simulink model "laser"  (R2017b)
settings: Solver=VariableStepAuto  StartTime=0.0  StopTime=10.0  RelTol=1e-3
values from neighbouring files (symbols this model uses):
  Amp0d = [1]    [System.m]    (also in System_submitted.m = [Amp0d1 Amp0d0])
  Amp0n = [1]    [System.m]    (also in System_submitted.m = Amp0n0)
  Amp1d = Amp0d    [System.m]    (also in SystemHeadless.m; System_submitted.m)
  Amp1n = Amp0n    [System.m]    (also in SystemHeadless.m; System_submitted.m)
  AmpSat0 = MotorParam(NomV)    [System.m]    (also in SystemHeadless.m = q0(NomV); System_submitted.m = q0(NomV))
  AmpSat1 = Big    [System.m]    (also in SystemHeadless.m = AmpSat0; System_submitted.m = AmpSat0)
  BackEMF0 = 1/K_B    [System.m]    (also in SystemHeadless.m = 1 / q0(SpdK); System_submitted.m = 1 / q0(SpdK))
  BackEMF1 = 1/K_B1    [System.m]    (also in SystemHeadless.m = 1 / q1(SpdK); System_submitted.m = 1 / q1(SpdK))
  Distance = 1    [CONSTANTS.m]
  Elec0d = [L_a R_a]    [System.m]    (also in SystemHeadless.m = [Elec0d1, Elec0d0]; System_submitted.m = [Elec0d1, Elec0d0])
  Elec0n = [1]    [System.m]    (also in SystemHeadless.m = 1; System_submitted.m = 1)
  Elec1d = [L_a R_a]    [System.m]    (also in SystemHeadless.m = [Elec1d1, Elec1d0]; System_submitted.m = [Elec1d1, Elec1d0])
  Elec1n = [1]    [System.m]    (also in SystemHeadless.m = 1; System_submitted.m = 1)
  JntSat1 = JntLim * RadPerDeg    [System.m]    (also in SystemHeadless.m = joint_limit; System_submitted.m = joint_limit)
  Mech0d = [J_system F_kf 0]    [System.m]    (also in SystemHeadless.m = [J_0, B_0, K_0]; System_submitted.m = [J_0, B_0, K_0])
  Mech0n = [1 0]    [System.m]    (also in SystemHeadless.m = [1, 0]; System_submitted.m = [1, 0])
  Mech1d = [J_rotor F_kf 0]    [System.m]    (also in SystemHeadless.m = [J_1, B_1, K_1]; System_submitted.m = [J_1, B_1, K_1])
  Mech1n = [1 0]    [System.m]    (also in SystemHeadless.m = [1, 0]; System_submitted.m = [1, 0])
  NomI0 = MotorParam(NomCurr)    [System.m]    (also in System_submitted.m = q0(NomCurr))
  NomI1 = MotorParam(NomCurr)    [System.m]    (also in System_submitted.m = q1(NomCurr))
  Sens0 = SensV / (SensAng * RadPerDeg)    [System.m]    (also in SystemHeadless.m; System_submitted.m)
  Sens1 = SensV / (SensAng * RadPerDeg)    [System.m]    (also in SystemHeadless.m; System_submitted.m)
  StallI0 = MotorParam(StallCurr)    [System.m]    (also in System_submitted.m = q0(StallCurr))
  StallI1 = MotorParam(StallCurr)    [System.m]    (also in System_submitted.m = q1(StallCurr))
  StFric0 = F_sf    [System.m]    (also in SystemHeadless.m = mu_SF * inner_fg; System_submitted.m = mu_SF * inner_fg)
  TConst0 = K_T    [System.m]    (also in SystemHeadless.m = q0(TorqueK); System_submitted.m = q0(TorqueK))
  TConst1 = K_T1    [System.m]    (also in SystemHeadless.m = q1(TorqueK); System_submitted.m = q1(TorqueK))
undefined symbols (not defined in the file or in its folder): FB0, FB1, PID0, PID1
libraries: simulink x11
settings Model: Creator=Moochster  LastModifiedBy=lucyl

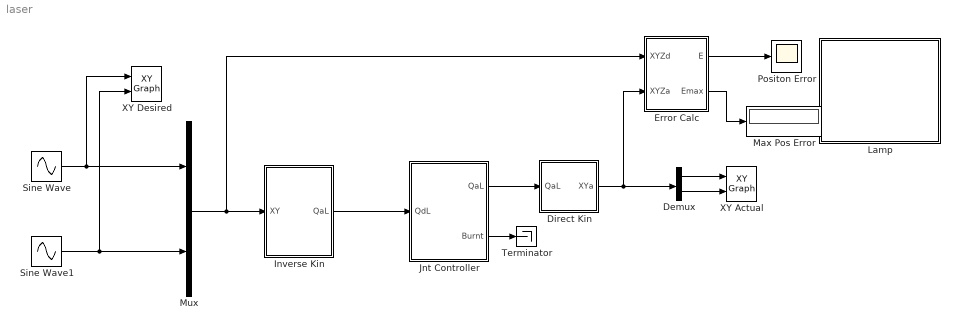
== system laser ==
  Demux : Demux  Outputs=2
  Direct Kin : Subsystem
  Error Calc : Subsystem
  Inverse Kin : Subsystem
  Jnt Controller : Subsystem
  Lamp : Subsystem  DialogController=hmiCreateDDGDialog  IsWebBlock=on  mask(MWDashboardBlock){webBlockId=7fcfd6b5-b98b-441a-9880-35fe4990fbef, webBlockType=lamp, ShowInLibBrowser=on, ShowInitialText=on, HMISrcModelName=laser}
      mask prompts: webBlockType "WebBlock Type"; HMISrcModelName "Source Model"
      mask help: SimulinkHMI:dialogs:LampDialogDesc
      mask Help: helpview([docroot '/mapfiles/simulink.map'], 'hmi_lamp')
      mask Display:
      | if strcmp(get_param(bdroot(gcb),'BlockDiagramType'), 'library')
      |     image([(matlabroot) '/toolbox/simulink/hmi/icons/Lamp.png']);
      | end
  Max Pos Error : Display
  Mux : Mux  Inputs=2
  Positon Error : Scope
  Sine Wave : Sin  Amplitude=50  SampleTime=0
  Sine Wave1 : Sin  Amplitude=50  Phase=pi/2  SampleTime=0
  Terminator : Terminator
  "XY Actual " : simulink/Sinks/XY Graph  xmin=-110  xmax=110  ymin=-110  ymax=110  st=-1
  XY Desired : simulink/Sinks/XY Graph  xmin=-110  xmax=110  ymin=-110  ymax=110  st=-1
  wires:
  Inverse Kin/1(QaL) -> Jnt Controller/1(QdL)
  Jnt Controller/1(QaL) -> Direct Kin/1(QaL)
  Mux/1 -> Error Calc/1(XYZd), Inverse Kin/1(XY)
  Sine Wave/1 -> XY Desired/1, Mux/1
  Sine Wave1/1 -> XY Desired/2, Mux/2
  Demux/2 -> "XY Actual "/2
  Demux/1 -> "XY Actual "/1
  Direct Kin/1(XYa) -> Error Calc/2(XYZa), Demux/1
  Error Calc/1(E) -> Positon Error/1
  Error Calc/2(Emax) -> Max Pos Error/1
  Jnt Controller/2(Burnt) -> Terminator/1

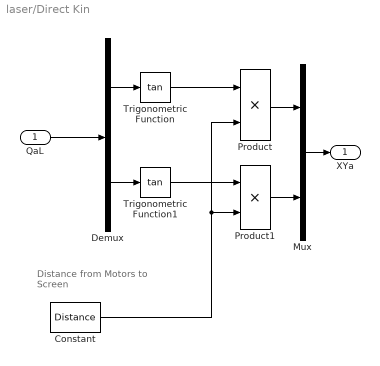
== system laser/Direct Kin ==
  note: Distance from Motors to Screen
  QaL : Inport
  Constant : Constant  Value=Distance
  Demux : Demux  Outputs=2
  Mux : Mux  Inputs=2
  Product : Product
  Product1 : Product
  Trigonometric Function : Trigonometry  Operator=tan
  Trigonometric Function1 : Trigonometry  Operator=tan
  XYa : Outport
  wires:
  QaL/1 -> Demux/1
  Mux/1 -> XYa/1
  Demux/1 -> Trigonometric Function/1
  Demux/2 -> Trigonometric Function1/1
  Trigonometric Function/1 -> Product/1
  Product/1 -> Mux/1
  Product1/1 -> Mux/2
  Trigonometric Function1/1 -> Product1/1
  Constant/1 -> Product/2, Product1/2

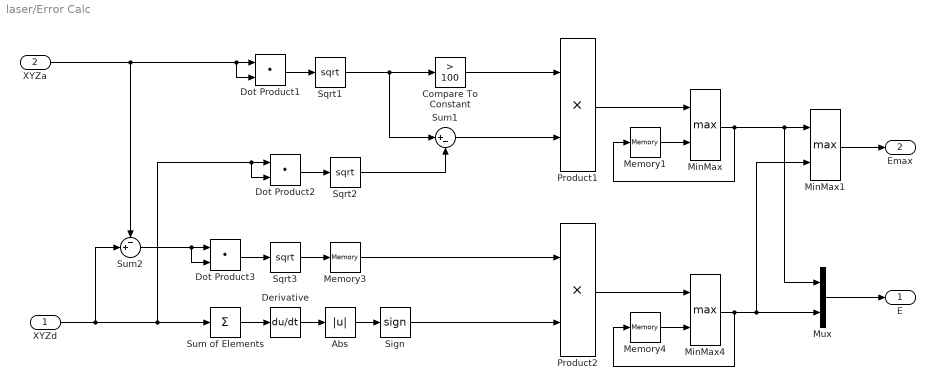
== system laser/Error Calc ==
  XYZd : Inport
  XYZa : Inport  Port=2
  Abs : Abs
  Compare To Constant : simulink/Logic and Bit Operations/Compare To Constant  relop=>  const=100  OutDataTypeStr=boolean
  Derivative : Derivative
  Dot Product1 : DotProduct  InputSameDT=on  OutDataTypeStr=Inherit: Inherit via internal rule
  Dot Product2 : DotProduct  InputSameDT=on  OutDataTypeStr=Inherit: Inherit via internal rule
  Dot Product3 : DotProduct  InputSameDT=on  OutDataTypeStr=Inherit: Inherit via internal rule
  Memory1 : Memory
  Memory3 : Memory
  Memory4 : Memory
  MinMax : MinMax  Function=max  Inputs=2
  MinMax1 : MinMax  Function=max  Inputs=2
  MinMax4 : MinMax  Function=max  Inputs=2
  Mux : Mux  Inputs=2
  Product1 : Product
  Product2 : Product
  Sign : Signum
  Sqrt1 : Sqrt  SaturateOnIntegerOverflow=on
  Sqrt2 : Sqrt  SaturateOnIntegerOverflow=on
  Sqrt3 : Sqrt  SaturateOnIntegerOverflow=on
  Sum of Elements : Sum  Inputs=+
  Sum1 : Sum  Inputs=|+-
  Sum2 : Sum  Inputs=-+|
  E : Outport
  Emax : Outport  Port=2
  wires:
  Sqrt3/1 -> Memory3/1
  Dot Product3/1 -> Sqrt3/1
  Sum2/1 -> Dot Product3/1, Dot Product3/2
  Sqrt2/1 -> Sum1/2
  Dot Product2/1 -> Sqrt2/1
  XYZd/1 -> Dot Product2/1, Dot Product2/2, Sum of Elements/1, Sum2/2
  Memory3/1 -> Product2/1
  Mux/1 -> E/1
  MinMax1/1 -> Emax/1
  MinMax4/1 -> Memory4/1, Mux/2, MinMax1/2
  Product2/1 -> MinMax4/1
  Memory4/1 -> MinMax4/2
  MinMax/1 -> Memory1/1, MinMax1/1, Mux/1
  Memory1/1 -> MinMax/2
  Sum1/1 -> Product1/2
  Compare To Constant/1 -> Product1/1
  Product1/1 -> MinMax/1
  Sqrt1/1 -> Compare To Constant/1, Sum1/1
  Sign/1 -> Product2/2
  Dot Product1/1 -> Sqrt1/1
  XYZa/1 -> Dot Product1/1, Dot Product1/2, Sum2/1
  Sum of Elements/1 -> Derivative/1
  Abs/1 -> Sign/1
  Derivative/1 -> Abs/1

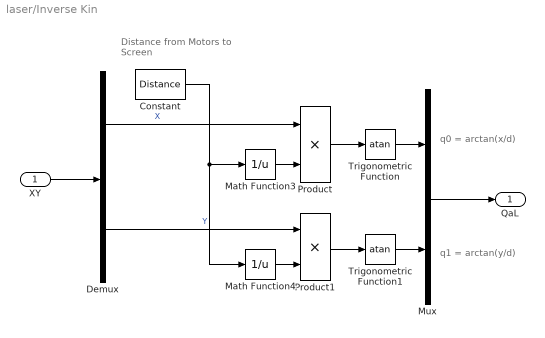
== system laser/Inverse Kin ==
  note: Distance from Motors to Screen
  note: q0 = arctan(x/d)
  note: q1 = arctan(y/d)
  XY : Inport
  Constant : Constant  Value=Distance
  Demux : Demux  Outputs=2
  Math Function3 : Math  Operator=reciprocal  SaturateOnIntegerOverflow=on
  Math Function4 : Math  Operator=reciprocal  SaturateOnIntegerOverflow=on
  Mux : Mux  Inputs=2
  Product : Product
  Product1 : Product
  Trigonometric Function : Trigonometry  Operator=atan
  Trigonometric Function1 : Trigonometry  Operator=atan
  QaL : Outport
  wires:
  XY/1 -> Demux/1
  Mux/1 -> QaL/1
  Demux/1 -> Product/1  "X"
  Demux/2 -> Product1/1  "Y"
  Trigonometric Function/1 -> Mux/1
  Trigonometric Function1/1 -> Mux/2
  Product/1 -> Trigonometric Function/1
  Product1/1 -> Trigonometric Function1/1
  Math Function3/1 -> Product/2
  Math Function4/1 -> Product1/2
  Constant/1 -> Math Function3/1, Math Function4/1

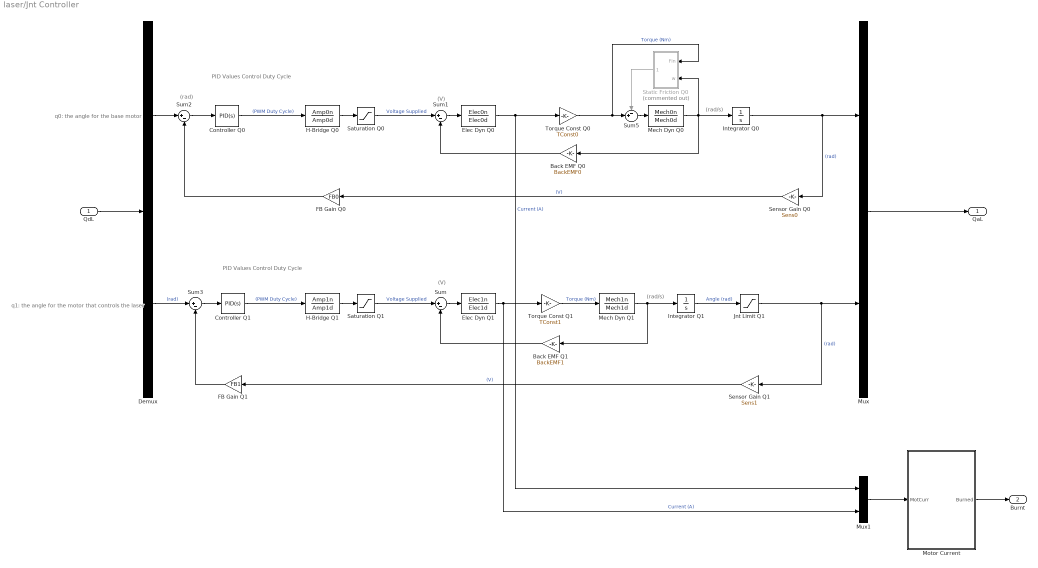
== system laser/Jnt Controller ==
  note: (rad/s)
  note: (V)
  note: (rad/s)
  note: (V)
  note: (rad)
  note: q0: the angle for the base motor
  note: q1: the angle for the motor that controls the laser
  note: PID Values Control Duty Cycle
  note: PID Values Control Duty Cycle
  QdL : Inport
  Back EMF Q0 : Gain  Gain=BackEMF0
  Back EMF Q1 : Gain  Gain=BackEMF1
  Controller Q0 : simulink/Continuous/PID Controller  Controller=PID  TimeDomain=Continuous-time  SampleTime=-1  IntegratorMethod=Forward Euler  FilterMethod=Forward Euler  Form=Parallel  UseFilter=on  ControllerParametersSource=internal  P=PID0(1)  I=PID0(2)  D=PID0(3)  N=100  InitialConditionSource=internal  InitialConditionForIntegrator=0  InitialConditionForFilter=0  ExternalReset=none  LimitOutput=off  UpperSaturationLimit=inf  LowerSaturationLimit=-inf  LinearizeAsGain=on  AntiWindupMode=none  Kb=1  TrackingMode=off  Kt=1  PParamMin=[]  PParamMax=[]  IParamMin=[]  IParamMax=[]  DParamMin=[]  DParamMax=[]  NParamMin=[]  NParamMax=[]  KbParamMin=[]  KbParamMax=[]  KtParamMin=[]  KtParamMax=[]  POutMin=[]  POutMax=[]  IOutMin=[]  IOutMax=[]  DOutMin=[]  DOutMax=[]  NOutMin=[]  NOutMax=[]  KbOutMin=[]  KbOutMax=[]  KtOutMin=[]  KtOutMax=[]  IntegratorOutMin=[]  IntegratorOutMax=[]  FilterOutMin=[]  FilterOutMax=[]  SumOutMin=[]  SumOutMax=[]  SumI1OutMin=[]  SumI1OutMax=[]  SumI2OutMin=[]  SumI2OutMax=[]  SumI3OutMin=[]  SumI3OutMax=[]  SumDOutMin=[]  SumDOutMax=[]  SaturationOutMin=[]  SaturationOutMax=[]  IntegratorContinuousStateAttributes=''  IntegratorStateMustResolveToSignalObject=off  IntegratorRTWStateStorageClass=Auto  FilterContinuousStateAttributes=''  FilterStateMustResolveToSignalObject=off  FilterRTWStateStorageClass=Auto  DifferentiatorICPrevScaledInput=0  DifferentiatorOutMin=[]  DifferentiatorOutMax=[]  InitialConditionSetting=State (most efficient)  FilterDiffOutCoefMin=[]  FilterDiffOutCoefMax=[]  SumDenOutMin=[]  SumDenOutMax=[]  SumNumOutMin=[]  SumNumOutMax=[]  ReciprocalOutMin=[]  ReciprocalOutMax=[]  DivideOutMin=[]  DivideOutMax=[]  TunerSelectOption=Transfer Function Based (PID Tuner App)
  Controller Q1 : simulink/Continuous/PID Controller  Controller=PID  TimeDomain=Continuous-time  SampleTime=-1  IntegratorMethod=Forward Euler  FilterMethod=Forward Euler  Form=Parallel  UseFilter=on  ControllerParametersSource=internal  P=PID1(1)  I=PID1(2)  D=PID1(3)  N=100  InitialConditionSource=internal  InitialConditionForIntegrator=0  InitialConditionForFilter=0  ExternalReset=none  LimitOutput=off  UpperSaturationLimit=inf  LowerSaturationLimit=-inf  LinearizeAsGain=on  AntiWindupMode=none  Kb=1  TrackingMode=off  Kt=1  PParamMin=[]  PParamMax=[]  IParamMin=[]  IParamMax=[]  DParamMin=[]  DParamMax=[]  NParamMin=[]  NParamMax=[]  KbParamMin=[]  KbParamMax=[]  KtParamMin=[]  KtParamMax=[]  POutMin=[]  POutMax=[]  IOutMin=[]  IOutMax=[]  DOutMin=[]  DOutMax=[]  NOutMin=[]  NOutMax=[]  KbOutMin=[]  KbOutMax=[]  KtOutMin=[]  KtOutMax=[]  IntegratorOutMin=[]  IntegratorOutMax=[]  FilterOutMin=[]  FilterOutMax=[]  SumOutMin=[]  SumOutMax=[]  SumI1OutMin=[]  SumI1OutMax=[]  SumI2OutMin=[]  SumI2OutMax=[]  SumI3OutMin=[]  SumI3OutMax=[]  SumDOutMin=[]  SumDOutMax=[]  SaturationOutMin=[]  SaturationOutMax=[]  IntegratorContinuousStateAttributes=''  IntegratorStateMustResolveToSignalObject=off  IntegratorRTWStateStorageClass=Auto  FilterContinuousStateAttributes=''  FilterStateMustResolveToSignalObject=off  FilterRTWStateStorageClass=Auto  DifferentiatorICPrevScaledInput=0  DifferentiatorOutMin=[]  DifferentiatorOutMax=[]  InitialConditionSetting=State (most efficient)  FilterDiffOutCoefMin=[]  FilterDiffOutCoefMax=[]  SumDenOutMin=[]  SumDenOutMax=[]  SumNumOutMin=[]  SumNumOutMax=[]  ReciprocalOutMin=[]  ReciprocalOutMax=[]  DivideOutMin=[]  DivideOutMax=[]  TunerSelectOption=Transfer Function Based (PID Tuner App)
  Demux : Demux  Outputs=2
  Elec Dyn Q0 : TransferFcn  Numerator=Elec0n  Denominator=Elec0d
  Elec Dyn Q1 : TransferFcn  Numerator=Elec1n  Denominator=Elec1d
  FB Gain Q0 : Gain  Gain=FB0
  FB Gain Q1 : Gain  Gain=FB1
  H-Bridge Q0 : TransferFcn  Numerator=Amp0n  Denominator=Amp0d
  H-Bridge Q1 : TransferFcn  Numerator=Amp1n  Denominator=Amp1d
  Integrator Q0 : Integrator
  Integrator Q1 : Integrator
  Jnt Limit Q1 : Saturate  UpperLimit=JntSat1  LowerLimit=-JntSat1
  Mech Dyn Q0 : TransferFcn  Numerator=Mech0n  Denominator=Mech0d
  Mech Dyn Q1 : TransferFcn  Numerator=Mech1n  Denominator=Mech1d
  Motor Current : Subsystem
  Mux : Mux  Inputs=2
  Mux1 : Mux  Inputs=2
  Saturation Q0 : Saturate  UpperLimit=AmpSat0  LowerLimit=-AmpSat0
  Saturation Q1 : Saturate  UpperLimit=AmpSat1  LowerLimit=-AmpSat1
  Sensor Gain Q0 : Gain  Gain=Sens0
  Sensor Gain Q1 : Gain  Gain=Sens1
  Static Friction Q0 : Subsystem  Commented=on
  Sum{,1..3} (4 alike) : Sum  Inputs=|+-
  Sum5 : Sum  Inputs=-+|
  Torque Const Q0 : Gain  Gain=TConst0
  Torque Const Q1 : Gain  Gain=TConst1
  QaL : Outport
  Burnt : Outport  Port=2
  wires:
  QdL/1 -> Demux/1
  Controller Q1/1 -> H-Bridge Q1/1  "(PWM Duty Cycle)"
  Sum/1 -> Elec Dyn Q1/1
  Sum3/1 -> Controller Q1/1
  Elec Dyn Q1/1 -> Mux1/2, Torque Const Q1/1  "Current (A)"
  H-Bridge Q1/1 -> Saturation Q1/1
  Back EMF Q1/1 -> Sum/2
  Controller Q0/1 -> H-Bridge Q0/1  "(PWM Duty Cycle)"
  Sum2/1 -> Controller Q0/1
  Elec Dyn Q0/1 -> Mux1/1, Torque Const Q0/1  "Current (A)"
  H-Bridge Q0/1 -> Saturation Q0/1
  Saturation Q0/1 -> Sum1/1  "Voltage Supplied"
  Back EMF Q0/1 -> Sum1/2
  Sum5/1 -> Mech Dyn Q0/1
  Jnt Limit Q1/1 -> Mux/2, Sensor Gain Q1/1  "(rad)"
  Demux/1 -> Sum2/1
  Demux/2 -> Sum3/1  "(rad)"
  FB Gain Q0/1 -> Sum2/2
  FB Gain Q1/1 -> Sum3/2
  Static Friction Q0/1(Fout) -> Sum5/1
  Torque Const Q1/1 -> Mech Dyn Q1/1  "Torque (Nm)"
  Sensor Gain Q1/1 -> FB Gain Q1/1  "(V)"
  Sensor Gain Q0/1 -> FB Gain Q0/1  "(V)"
  Mech Dyn Q0/1 -> Static Friction Q0/2(w), Integrator Q0/1, Back EMF Q0/1
  Integrator Q0/1 -> Sensor Gain Q0/1, Mux/1  "(rad)"
  Integrator Q1/1 -> Jnt Limit Q1/1  "Angle (rad)"
  Torque Const Q0/1 -> Static Friction Q0/1(Fin), Sum5/2  "Torque (Nm)"
  Mech Dyn Q1/1 -> Integrator Q1/1, Back EMF Q1/1
  Sum1/1 -> Elec Dyn Q0/1
  Saturation Q1/1 -> Sum/1  "Voltage Supplied"
  Mux/1 -> QaL/1
  Mux1/1 -> Motor Current/1(MotCurr)
  Motor Current/1(Burned) -> Burnt/1

== system laser/Lamp ==

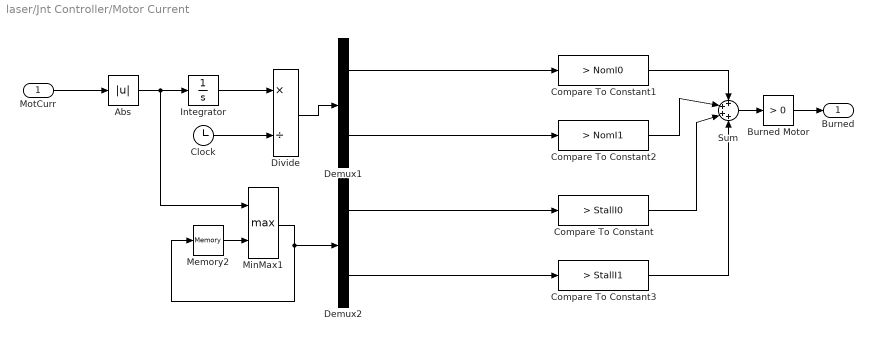
== system laser/Jnt Controller/Motor Current ==
  MotCurr : Inport
  Abs : Abs
  Burned Motor : simulink/Logic and Bit Operations/Compare To Zero  relop=>  OutDataTypeStr=boolean
  Clock : Clock
  Compare To Constant : simulink/Logic and Bit Operations/Compare To Constant  relop=>  const=StallI0  OutDataTypeStr=boolean
  Compare To Constant1 : simulink/Logic and Bit Operations/Compare To Constant  relop=>  const=NomI0  OutDataTypeStr=boolean
  Compare To Constant2 : simulink/Logic and Bit Operations/Compare To Constant  relop=>  const=NomI1  OutDataTypeStr=boolean
  Compare To Constant3 : simulink/Logic and Bit Operations/Compare To Constant  relop=>  const=StallI1  OutDataTypeStr=boolean
  Demux1 : Demux  Outputs=2
  Demux2 : Demux  Outputs=2
  Divide : Product  Inputs=*/
  Integrator : Integrator
  Memory2 : Memory
  MinMax1 : MinMax  Function=max  Inputs=2
  Sum : Sum  Inputs=++++
  Burned : Outport
  wires:
  Sum/1 -> Burned Motor/1
  Burned Motor/1 -> Burned/1
  MinMax1/1 -> Memory2/1, Demux2/1
  Memory2/1 -> MinMax1/2
  Compare To Constant2/1 -> Sum/2
  Compare To Constant/1 -> Sum/3
  Compare To Constant3/1 -> Sum/4
  Compare To Constant1/1 -> Sum/1
  Demux2/2 -> Compare To Constant3/1
  Demux1/2 -> Compare To Constant2/1
  Demux2/1 -> Compare To Constant/1
  Abs/1 -> Integrator/1, MinMax1/1
  Divide/1 -> Demux1/1
  Clock/1 -> Divide/2
  Integrator/1 -> Divide/1
  MotCurr/1 -> Abs/1
  Demux1/1 -> Compare To Constant1/1

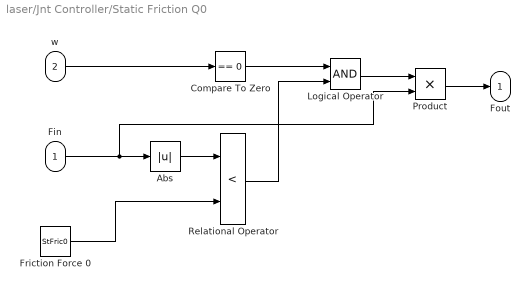
== system laser/Jnt Controller/Static Friction Q0 ==
  Fin : Inport
  w : Inport  Port=2
  Abs : Abs
  Compare To Zero : simulink/Logic and Bit Operations/Compare To Zero  relop===  OutDataTypeStr=boolean
  Friction Force 0 : Constant  Value=StFric0
  Logical Operator : Logic  AllPortsSameDT=off  OutDataTypeStr=boolean
  Product : Product
  Relational Operator : RelationalOperator  Operator=<  OutDataTypeStr=boolean  RndMeth=Simplest
  Fout : Outport
  wires:
  Friction Force 0/1 -> Relational Operator/2
  Product/1 -> Fout/1
  Compare To Zero/1 -> Logical Operator/1
  Relational Operator/1 -> Logical Operator/2
  Logical Operator/1 -> Product/1
  Fin/1 -> Product/2, Abs/1
  w/1 -> Compare To Zero/1
  Abs/1 -> Relational Operator/1
